simulink model "SFEnum_PP"  (R2017b)
settings: Solver=FixedStepDiscrete  StartTime=0.0  StopTime=10.0  FixedStep=1.000000  RelTol=1e-3
model workspace (MAT data in the model file):
  ContractValidatorBlocksMap = containers.Map
  ContractValidatorBlocksMap.serialization.keys = {'DaysEnum/contract/validator', 'days/contract/validator'}
  ContractValidatorBlocksMap.serialization.values{1}.block = 'DaysEnum/contract/validator'
  ContractValidatorBlocksMap.serialization.values{1}.assumePorts = 0
  ContractValidatorBlocksMap.serialization.values{1}.guaranteePorts = 1
  ContractValidatorBlocksMap.serialization.values{1}.modeBlocksPorts = 0
  ContractValidatorBlocksMap.serialization.values{1}.portHandles.Inport = 64.0010986328
  ContractValidatorBlocksMap.serialization.values{1}.portHandles.Outport = 65.0003662109
  ContractValidatorBlocksMap.serialization.values{1}.portHandles.Enable = []
  ContractValidatorBlocksMap.serialization.values{1}.portHandles.Trigger = []
  ContractValidatorBlocksMap.serialization.values{1}.portHandles.State = []
  ContractValidatorBlocksMap.serialization.values{1}.portHandles.LConn = []
  ContractValidatorBlocksMap.serialization.values{1}.portHandles.RConn = []
  ContractValidatorBlocksMap.serialization.values{1}.portHandles.Ifaction = []
  ContractValidatorBlocksMap.serialization.values{1}.portHandles.Reset = []
  ContractValidatorBlocksMap.serialization.values{1}.portConnectivity(1).Type = '1'
  ContractValidatorBlocksMap.serialization.values{1}.portConnectivity(1).Position = [375 75]
  ContractValidatorBlocksMap.serialization.values{1}.portConnectivity(1).SrcBlock = 10.0003662109
  ContractValidatorBlocksMap.serialization.values{1}.portConnectivity(1).SrcPort = 0
  ContractValidatorBlocksMap.serialization.values{1}.portConnectivity(1).DstBlock = []
  ContractValidatorBlocksMap.serialization.values{1}.portConnectivity(1).DstPort = []
  ContractValidatorBlocksMap.serialization.values{1}.portConnectivity(2).Type = '1'
  ContractValidatorBlocksMap.serialization.values{1}.portConnectivity(2).Position = [505 75]
  ContractValidatorBlocksMap.serialization.values{1}.portConnectivity(2).SrcBlock = []
  ContractValidatorBlocksMap.serialization.values{1}.portConnectivity(2).SrcPort = []
  ContractValidatorBlocksMap.serialization.values{1}.portConnectivity(2).DstBlock = 35.0003662109
  ContractValidatorBlocksMap.serialization.values{1}.portConnectivity(2).DstPort = 0
  ContractValidatorBlocksMap.serialization.values{2}.block = 'days/contract/validator'
  ContractValidatorBlocksMap.serialization.values{2}.assumePorts = 0
  ContractValidatorBlocksMap.serialization.values{2}.guaranteePorts = 1
  ContractValidatorBlocksMap.serialization.values{2}.modeBlocksPorts = 0
  ContractValidatorBlocksMap.serialization.values{2}.portHandles.Inport = 174.00012207
  ContractValidatorBlocksMap.serialization.values{2}.portHandles.Outport = 168.000366211
  ContractValidatorBlocksMap.serialization.values{2}.portHandles.Enable = []
  ContractValidatorBlocksMap.serialization.values{2}.portHandles.Trigger = []
  ContractValidatorBlocksMap.serialization.values{2}.portHandles.State = []
  ContractValidatorBlocksMap.serialization.values{2}.portHandles.LConn = []
  ContractValidatorBlocksMap.serialization.values{2}.portHandles.RConn = []
  ContractValidatorBlocksMap.serialization.values{2}.portHandles.Ifaction = []
  ContractValidatorBlocksMap.serialization.values{2}.portHandles.Reset = []
  ContractValidatorBlocksMap.serialization.values{2}.portConnectivity(1).Type = '1'
  ContractValidatorBlocksMap.serialization.values{2}.portConnectivity(1).Position = [375 75]
  ContractValidatorBlocksMap.serialization.values{2}.portConnectivity(1).SrcBlock = 290.00012207
  ContractValidatorBlocksMap.serialization.values{2}.portConnectivity(1).SrcPort = 0
  ContractValidatorBlocksMap.serialization.values{2}.portConnectivity(1).DstBlock = []
  ContractValidatorBlocksMap.serialization.values{2}.portConnectivity(1).DstPort = []
  ContractValidatorBlocksMap.serialization.values{2}.portConnectivity(2).Type = '1'
  ContractValidatorBlocksMap.serialization.values{2}.portConnectivity(2).Position = [505 75]
  ContractValidatorBlocksMap.serialization.values{2}.portConnectivity(2).SrcBlock = []
  ContractValidatorBlocksMap.serialization.values{2}.portConnectivity(2).SrcPort = []
  ContractValidatorBlocksMap.serialization.values{2}.portConnectivity(2).DstBlock = 152.00012207
  ContractValidatorBlocksMap.serialization.values{2}.portConnectivity(2).DstPort = 0
  ContractValidatorBlocksMap.serialization.uniformity = 0
  ContractValidatorBlocksMap.serialization.keyType = 'char'
  ContractValidatorBlocksMap.serialization.valueType = 'any'
  already_pp = 1
undefined symbols (not defined in the file): Days
settings Model: Creator=mudat  LastModifiedBy=hbourbou
settings DebuggingCC: AlgebraicLoopMsg=error  ArtificialAlgebraicLoopMsg=error  SingleTaskRateTransMsg=error
settings CodeAppCC: StateflowObjectComments=on

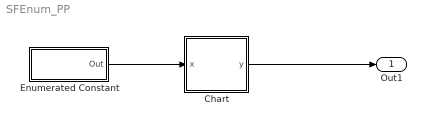
== system SFEnum_PP ==
  Chart : Stateflow chart  TreatAsAtomicUnit=on
  Enumerated Constant : Subsystem  AncestorBlock=simulink/Sources/Enumerated Constant  DialogController=Simulink.DDGSource  TreatAsAtomicUnit=on  mask(Enumerated Constant){OutDataTypeStr=Enum: Days, Value=Days.Saturday, SampleTime=inf}
      mask prompts: OutDataTypeStr "Simulink:blkprm_prompts:OutputDataType"; Value "Simulink:blkprm_prompts:ConstConstValue"; SampleTime "Simulink:blkprm_prompts:AllSrcBlksSampleTime"
      mask init:
      | % Check data type & value
      | enumconst_cb('MaskInit', get_param(gcb, 'OutDataTypeStr'), Value);
      mask TypeOptions SampleTime: Constant/SampleTime
      mask Display:
      | % Get string to use for display purposes
      | enumConstDispStr = get_param(gcbh, 'Value');
      | if isempty(enumConstDispStr)
      |   enumConstDispStr = '???';
      | end
      | disp(enumConstDispStr)
  Out1 : Outport
  wires:
  Enumerated Constant/1(Out) -> Chart/1(x)
  Chart/1(y) -> Out1/1

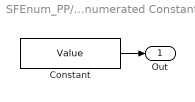
== system SFEnum_PP/Enumerated Constant ==
  Constant : Constant  DialogController=Simulink.DDGSource  Value=Value  OutDataTypeStr=OutDataTypeStr  SampleTime=SampleTime  LockScale=on
  Out : Outport  OutDataTypeStr=OutDataTypeStr
  wires:
  Constant/1 -> Out/1

== stateflow chart SFEnum_PP/Chart ==
  state A_
    en, du: y = x;
  (default) -> A_
  data: x input Enum: Days; y output Enum: Days
